simulink model "gpc_simulink"  (R2022a)
settings: Solver=VariableStepAuto  StartTime=0.0  StopTime=20  RelTol=1e-3
values from neighbouring files (symbols this model uses):
  H = inv(G'*G+lambda*eye(3))    [gpc.m]
  K = inv(G'*G+lambda*eye(3))*G'    [gpc.m]
  th = 1    [gpc.m]
undefined symbols (not defined in the file or in its folder): DiscIntNeverNeededParam
libraries: ctrlSharedLib x5, eeAlternativeControllers x1, slident x1
settings Model: Creator=mjwhi  LastModifiedBy=mjwhi

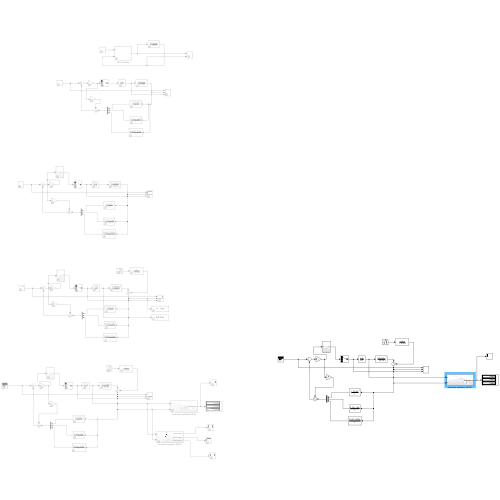
[thumbnail: Simulink's stored preview of the top-level diagram]
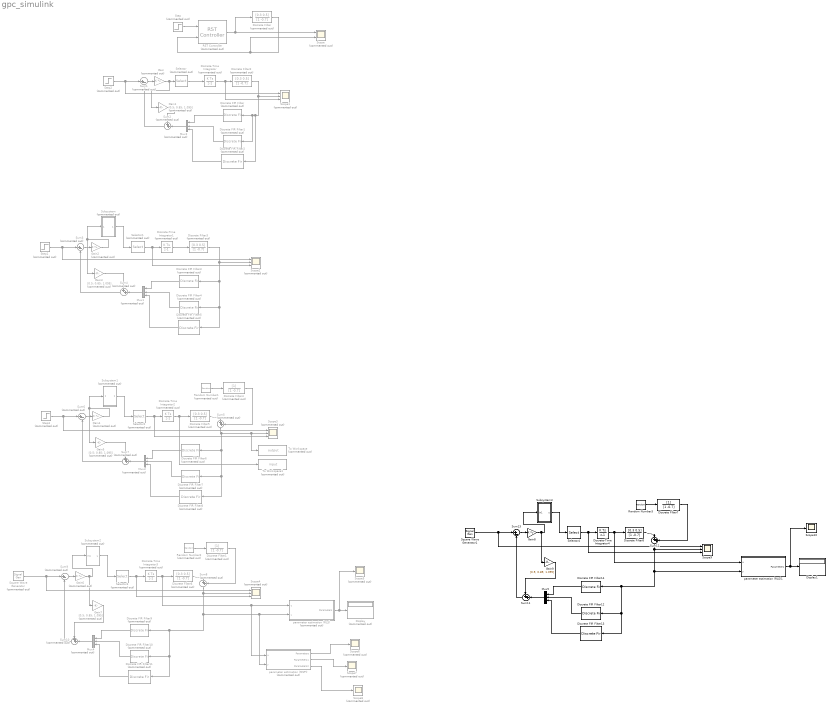
== system gpc_simulink ==
  Discrete FIR Filter{,3,6,9} (4 alike) : DiscreteFir  Commented=on  Coefficients=[1.7 -0.7]
  Discrete FIR Filter{1,4,7,10} (4 alike) : DiscreteFir  Commented=on  Coefficients=[2.19 -1.19]
  Discrete FIR Filter{2,5,8,11} (4 alike) : DiscreteFir  Commented=on  Coefficients=[2.533 -1.533]
  Discrete FIR Filter12 : DiscreteFir  Coefficients=[2.19 -1.19]
  Discrete FIR Filter13 : DiscreteFir  Coefficients=[2.533 -1.533]
  Discrete FIR Filter14 : DiscreteFir  Coefficients=[1.7 -0.7]
  Discrete Filter{,2..3,5} (4 alike) : DiscreteFilter  Commented=on  Numerator=[0.3 0.5]  Denominator=[1 -0.7]
  Discrete Filter1 : DiscreteFilter  Commented=on  Denominator=[1 -0.7]
  Discrete Filter4 : DiscreteFilter  Commented=on  Denominator=[1 -0.7]
  Discrete Filter6 : DiscreteFilter  Commented=on  Numerator=[0.3 0.5]  Denominator=[1 -0.7]  InitialStates=1
  Discrete Filter7 : DiscreteFilter  Denominator=[1 -0.7]
  Discrete Filter8 : DiscreteFilter  Numerator=[0.3 0.5]  Denominator=[1 -0.7]  InitialStates=1
  Discrete-Time Integrator{,1..3} (4 alike) : DiscreteIntegrator  Commented=on  SampleTime=-1  ICPrevOutput=DiscIntNeverNeededParam  ICPrevScaledInput=DiscIntNeverNeededParam
  Discrete-Time Integrator4 : DiscreteIntegrator  SampleTime=-1  ICPrevOutput=DiscIntNeverNeededParam  ICPrevScaledInput=DiscIntNeverNeededParam
  Display : Display  Commented=on
  Display1 : Display
  Gain{,2,4,6} (4 alike) : Gain  Commented=on  Gain=K  Multiplication=Matrix(K*u)
  Gain{1,3,5,7} (4 alike) : Gain  Commented=on  Gain=[0.5; 0.85; 1.095]
  Gain8 : Gain  Gain=K  Multiplication=Matrix(K*u)
  Gain9 : Gain  Gain=[0.5; 0.85; 1.095]
  Mux{1..4} (4 alike) : Mux  Commented=on  Inputs=3
  Mux5 : Mux  Inputs=3
  RST Controller : eeAlternativeControllers/RST Controller  Commented=on  CtrlParam=Generate polynomials  R=1  S=1  T=1  B=[0.3 0.5]  A=[1 -0.7]  N=3  lam=0.7  d=0  Ts=-1
      settings: SourceProductBaseCode=PS
  Random Number1 : RandomNumber  Commented=on  Variance=0.001  SampleTime=0.2
  Random Number2 : RandomNumber  Commented=on  Variance=0.001  SampleTime=0.2
  Random Number3 : RandomNumber  Variance=0.001  SampleTime=0.2
  Scope : Scope  Commented=on  NumInputPorts=2
  Scope{1..4} (4 alike) : Scope  Commented=on  NumInputPorts=3
  Scope10 : Scope
  Scope{5..8} (4 alike) : Scope  Commented=on
  Scope9 : Scope  NumInputPorts=3
  Selector{,1..3} (4 alike) : Selector  Commented=on  InputPortWidth=3  IndexOptions=Index vector (dialog)  Indices=[1]  OutputSizes=1
  Selector4 : Selector  InputPortWidth=3  IndexOptions=Index vector (dialog)  Indices=[1]  OutputSizes=1
  Square Wave Generator : SignalGenerator  Commented=on  WaveForm=square  Units=rad/sec
  Square Wave Generator1 : SignalGenerator  WaveForm=square  Units=rad/sec
  Step{,1..3} (4 alike) : Step  Commented=on  Time=0  SampleTime=0.2
  Subsystem : Subsystem  Commented=on
  Subsystem1 : Subsystem  Commented=on
  Subsystem2 : Subsystem  Commented=on
  Subsystem3 : Subsystem
  Sum{1,3,6,9} (4 alike) : Sum  Commented=on  Inputs=|+-
  Sum{2,4,7,10} (4 alike) : Sum  Commented=on  Inputs=++|
  Sum11 : Sum  Inputs=++|
  Sum12 : Sum  Inputs=|++
  Sum13 : Sum  Inputs=|+-
  Sum5 : Sum  Commented=on  Inputs=|++
  Sum8 : Sum  Commented=on  Inputs=|++
  To Workspace : ToWorkspace  Commented=on  VariableName=output  SaveFormat=Timeseries  SampleTime=-1
  To Workspace1 : ToWorkspace  Commented=on  VariableName=input  SaveFormat=Timeseries  SampleTime=-1
  parameter estimation (MSPI) : Subsystem  Commented=on
  parameter estimation (RLS) : Subsystem  Commented=on
  parameter estimation (RLS)1 : Subsystem
  wires:
  RST Controller/1 -> Discrete Filter/1, Scope/1
  Step/1 -> RST Controller/1
  Discrete Filter/1 -> Scope/2, RST Controller/2
  Sum1/1 -> Gain/1
  Sum2/1 -> Sum1/2
  Step2/1 -> Scope1/1, Sum1/1
  Gain/1 -> Gain1/1, Selector/1
  Gain1/1 -> Sum2/1
  Discrete Filter2/1 -> Discrete FIR Filter2/1, Discrete FIR Filter1/1, Discrete FIR Filter/1, Scope1/2
  Discrete FIR Filter/1 -> Mux2/1
  Discrete FIR Filter1/1 -> Mux2/2
  Discrete FIR Filter2/1 -> Mux2/3
  Mux2/1 -> Sum2/2
  Selector/1 -> Discrete-Time Integrator/1
  Discrete-Time Integrator/1 -> Scope1/3, Discrete Filter2/1
  Selector1/1 -> Scope2/3, Discrete-Time Integrator1/1
  Discrete-Time Integrator1/1 -> Discrete Filter3/1
  Mux1/1 -> Sum4/2
  Discrete FIR Filter5/1 -> Mux1/3
  Step1/1 -> Scope2/1, Sum3/1
  Gain3/1 -> Sum4/1
  Discrete FIR Filter3/1 -> Mux1/1
  Discrete FIR Filter4/1 -> Mux1/2
  Sum3/1 -> Gain2/1
  Gain2/1 -> Gain3/1, Subsystem/1(In1)
  Sum4/1 -> Sum3/2
  Subsystem/1(Out1) -> Selector1/1
  Discrete Filter3/1 -> Discrete FIR Filter4/1, Discrete FIR Filter5/1, Discrete FIR Filter3/1, Scope2/2
  Sum6/1 -> Gain4/1
  Discrete FIR Filter7/1 -> Mux3/2
  Discrete FIR Filter6/1 -> Mux3/1
  Discrete FIR Filter8/1 -> Mux3/3
  Gain5/1 -> Sum7/1
  Mux3/1 -> Sum7/2
  Step3/1 -> Scope3/1, Sum6/1
  Discrete-Time Integrator2/1 -> To Workspace1/1, Discrete Filter5/1
  Discrete Filter5/1 -> Sum5/1
  Sum7/1 -> Sum6/2
  Discrete Filter4/1 -> Sum5/2
  Sum5/1 -> Discrete FIR Filter7/1, Discrete FIR Filter8/1, Discrete FIR Filter6/1, Scope3/2, To Workspace/1
  Selector2/1 -> Scope3/3, Discrete-Time Integrator2/1
  Subsystem1/1(Out1) -> Selector2/1
  Random Number1/1 -> Discrete Filter4/1
  Gain4/1 -> Gain5/1, Subsystem1/1(In1)
  Subsystem2/1(u) -> Selector3/1
  Selector3/1 -> Scope4/3, Discrete-Time Integrator3/1
  Square Wave Generator/1 -> Scope4/1, Sum9/1
  Random Number2/1 -> Discrete Filter1/1
  Discrete-Time Integrator3/1 -> parameter estimation (RLS)/1(u), parameter estimation (MSPI)/1(u), Discrete Filter6/1
  Gain6/1 -> Gain7/1, Subsystem2/1(In1)
  Discrete Filter6/1 -> Sum8/1
  Sum9/1 -> Gain6/1
  Discrete Filter1/1 -> Sum8/2
  parameter estimation (RLS)/1(Parameters) -> Scope5/1, Display/1
  Sum8/1 -> Scope4/2, Discrete FIR Filter10/1, Discrete FIR Filter11/1, Discrete FIR Filter9/1, parameter estimation (RLS)/2(y), parameter estimation (MSPI)/2(y)
  Mux4/1 -> Sum10/2
  Sum10/1 -> Sum9/2
  Discrete FIR Filter11/1 -> Mux4/3
  Gain7/1 -> Sum10/1
  Discrete FIR Filter9/1 -> Mux4/1
  Discrete FIR Filter10/1 -> Mux4/2
  parameter estimation (MSPI)/1(Parameters) -> Scope6/1
  parameter estimation (MSPI)/2(Parameters1) -> Scope7/1
  parameter estimation (MSPI)/3(Parameters2) -> Scope8/1
  Sum11/1 -> Sum13/2
  Discrete FIR Filter14/1 -> Mux5/1
  Discrete FIR Filter12/1 -> Mux5/2
  Mux5/1 -> Sum11/2
  parameter estimation (RLS)1/1(Parameters) -> Scope10/1, Display1/1
  Gain9/1 -> Sum11/1
  Sum12/1 -> Scope9/2, Discrete FIR Filter12/1, Discrete FIR Filter13/1, Discrete FIR Filter14/1, parameter estimation (RLS)1/2(y)
  Discrete Filter7/1 -> Sum12/2
  Gain8/1 -> Gain9/1, Subsystem3/1(In1)
  Discrete-Time Integrator4/1 -> parameter estimation (RLS)1/1(u), Discrete Filter8/1
  Discrete FIR Filter13/1 -> Mux5/3
  Random Number3/1 -> Discrete Filter7/1
  Sum13/1 -> Gain8/1
  Discrete Filter8/1 -> Sum12/1
  Square Wave Generator1/1 -> Scope9/1, Sum13/1
  Subsystem3/1(u) -> Selector4/1
  Selector4/1 -> Scope9/3, Discrete-Time Integrator4/1

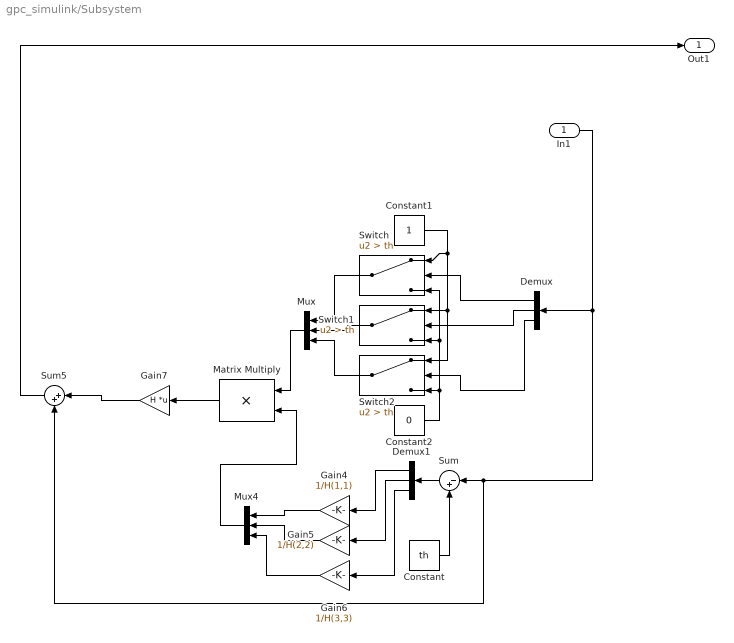
== system gpc_simulink/Subsystem ==
  In1 : Inport
  Constant : Constant  Value=th
  Constant1 : Constant
  Constant2 : Constant  Value=0
  Demux : Demux  Outputs=3
  Demux1 : Demux  Outputs=3
  Gain4 : Gain  Gain=1/H(1,1)
  Gain5 : Gain  Gain=1/H(2,2)
  Gain6 : Gain  Gain=1/H(3,3)
  Gain7 : Gain  Gain=H  Multiplication=Matrix(K*u)
  Matrix Multiply : Product
  Mux : Mux  Inputs=3
  Mux4 : Mux  Inputs=3
  Sum : Sum  Inputs=|-+
  Sum5 : Sum  Inputs=|++
  Switch : Switch  Criteria=u2 > Threshold  Threshold=th  SaturateOnIntegerOverflow=off  InputSameDT=off
  Switch1 : Switch  Criteria=u2 > Threshold  Threshold=th  SaturateOnIntegerOverflow=off  InputSameDT=off
  Switch2 : Switch  Criteria=u2 > Threshold  Threshold=th  SaturateOnIntegerOverflow=off  InputSameDT=off
  Out1 : Outport
  wires:
  Mux4/1 -> Matrix Multiply/2
  Demux/3 -> Switch2/2
  Constant2/1 -> Switch/3, Switch1/3, Switch2/3
  In1/1 -> Sum5/2, Sum/1, Demux/1
  Mux/1 -> Matrix Multiply/1
  Constant1/1 -> Switch/1, Switch2/1, Switch1/1
  Sum/1 -> Demux1/1
  Gain4/1 -> Mux4/1
  Demux1/3 -> Gain6/1
  Constant/1 -> Sum/2
  Gain7/1 -> Sum5/1
  Demux/1 -> Switch/2
  Gain5/1 -> Mux4/2
  Demux/2 -> Switch1/2
  Matrix Multiply/1 -> Gain7/1
  Switch/1 -> Mux/1
  Switch1/1 -> Mux/2
  Demux1/2 -> Gain5/1
  Switch2/1 -> Mux/3
  Demux1/1 -> Gain4/1
  Gain6/1 -> Mux4/3
  Sum5/1 -> Out1/1

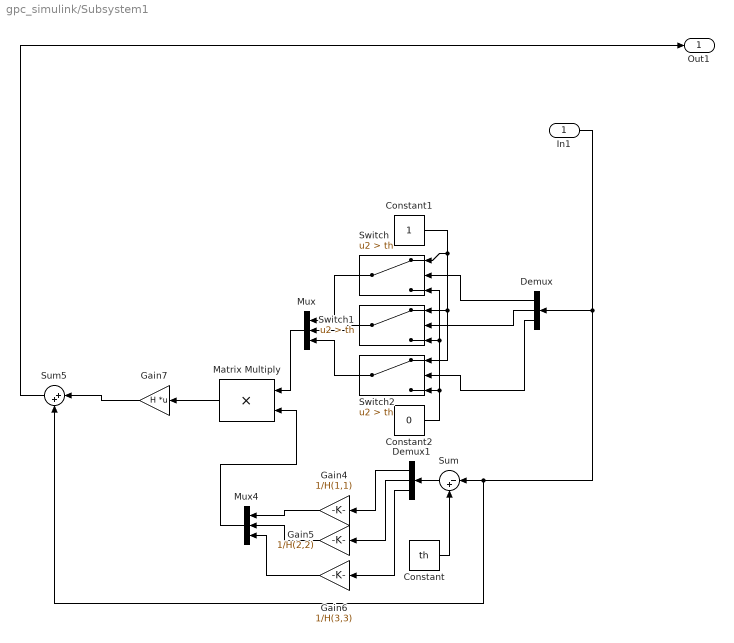
== system gpc_simulink/Subsystem1 ==
  In1 : Inport
  Constant : Constant  Value=th
  Constant1 : Constant
  Constant2 : Constant  Value=0
  Demux : Demux  Outputs=3
  Demux1 : Demux  Outputs=3
  Gain4 : Gain  Gain=1/H(1,1)
  Gain5 : Gain  Gain=1/H(2,2)
  Gain6 : Gain  Gain=1/H(3,3)
  Gain7 : Gain  Gain=H  Multiplication=Matrix(K*u)
  Matrix Multiply : Product
  Mux : Mux  Inputs=3
  Mux4 : Mux  Inputs=3
  Sum : Sum  Inputs=|-+
  Sum5 : Sum  Inputs=|++
  Switch : Switch  Criteria=u2 > Threshold  Threshold=th  SaturateOnIntegerOverflow=off  InputSameDT=off
  Switch1 : Switch  Criteria=u2 > Threshold  Threshold=th  SaturateOnIntegerOverflow=off  InputSameDT=off
  Switch2 : Switch  Criteria=u2 > Threshold  Threshold=th  SaturateOnIntegerOverflow=off  InputSameDT=off
  Out1 : Outport
  wires:
  Mux4/1 -> Matrix Multiply/2
  Demux/3 -> Switch2/2
  Constant2/1 -> Switch/3, Switch1/3, Switch2/3
  In1/1 -> Sum5/2, Sum/1, Demux/1
  Mux/1 -> Matrix Multiply/1
  Constant1/1 -> Switch/1, Switch2/1, Switch1/1
  Sum/1 -> Demux1/1
  Gain4/1 -> Mux4/1
  Demux1/3 -> Gain6/1
  Constant/1 -> Sum/2
  Gain7/1 -> Sum5/1
  Demux/1 -> Switch/2
  Gain5/1 -> Mux4/2
  Demux/2 -> Switch1/2
  Matrix Multiply/1 -> Gain7/1
  Switch/1 -> Mux/1
  Switch1/1 -> Mux/2
  Demux1/2 -> Gain5/1
  Switch2/1 -> Mux/3
  Demux1/1 -> Gain4/1
  Gain6/1 -> Mux4/3
  Sum5/1 -> Out1/1

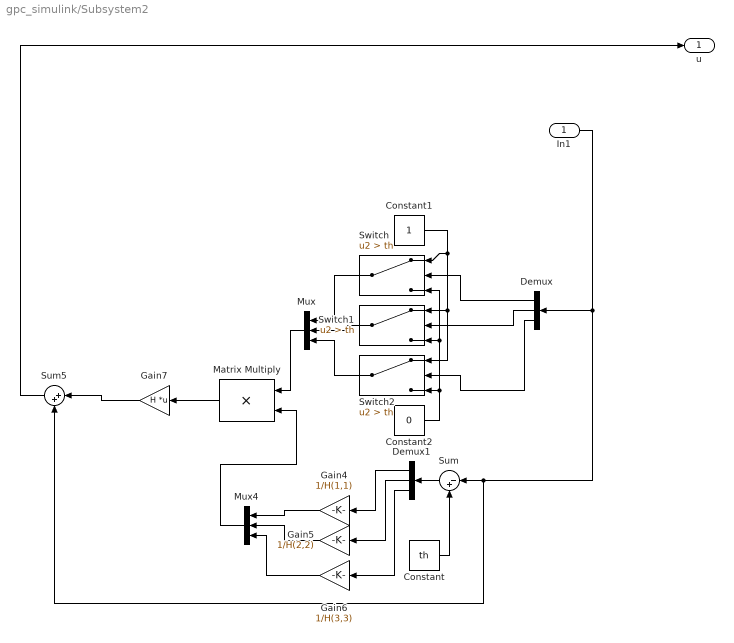
== system gpc_simulink/Subsystem2 ==
  In1 : Inport
  Constant : Constant  Value=th
  Constant1 : Constant
  Constant2 : Constant  Value=0
  Demux : Demux  Outputs=3
  Demux1 : Demux  Outputs=3
  Gain4 : Gain  Gain=1/H(1,1)
  Gain5 : Gain  Gain=1/H(2,2)
  Gain6 : Gain  Gain=1/H(3,3)
  Gain7 : Gain  Gain=H  Multiplication=Matrix(K*u)
  Matrix Multiply : Product
  Mux : Mux  Inputs=3
  Mux4 : Mux  Inputs=3
  Sum : Sum  Inputs=|-+
  Sum5 : Sum  Inputs=|++
  Switch : Switch  Criteria=u2 > Threshold  Threshold=th  SaturateOnIntegerOverflow=off  InputSameDT=off
  Switch1 : Switch  Criteria=u2 > Threshold  Threshold=th  SaturateOnIntegerOverflow=off  InputSameDT=off
  Switch2 : Switch  Criteria=u2 > Threshold  Threshold=th  SaturateOnIntegerOverflow=off  InputSameDT=off
  u : Outport
  wires:
  Mux4/1 -> Matrix Multiply/2
  Demux/3 -> Switch2/2
  Constant2/1 -> Switch/3, Switch1/3, Switch2/3
  In1/1 -> Sum5/2, Sum/1, Demux/1
  Mux/1 -> Matrix Multiply/1
  Constant1/1 -> Switch/1, Switch2/1, Switch1/1
  Sum/1 -> Demux1/1
  Gain4/1 -> Mux4/1
  Demux1/3 -> Gain6/1
  Constant/1 -> Sum/2
  Gain7/1 -> Sum5/1
  Demux/1 -> Switch/2
  Gain5/1 -> Mux4/2
  Demux/2 -> Switch1/2
  Matrix Multiply/1 -> Gain7/1
  Switch/1 -> Mux/1
  Switch1/1 -> Mux/2
  Demux1/2 -> Gain5/1
  Switch2/1 -> Mux/3
  Demux1/1 -> Gain4/1
  Gain6/1 -> Mux4/3
  Sum5/1 -> u/1

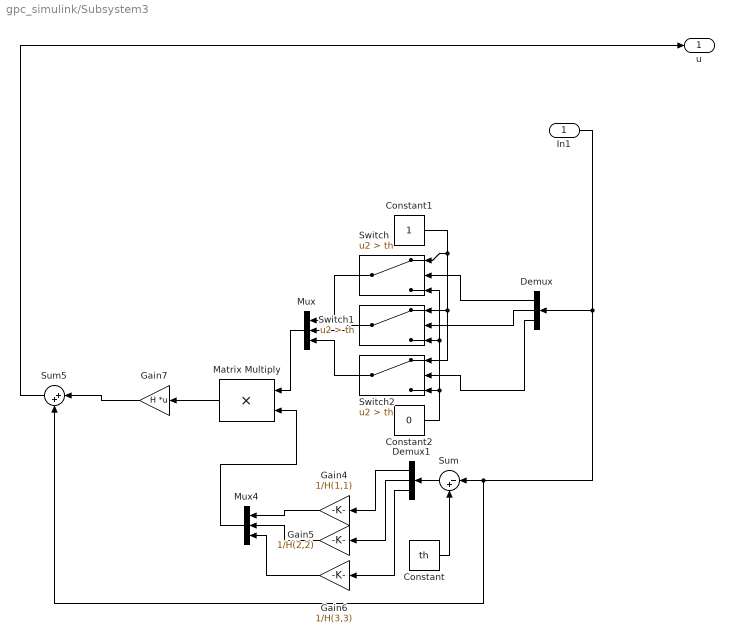
== system gpc_simulink/Subsystem3 ==
  In1 : Inport
  Constant : Constant  Value=th
  Constant1 : Constant
  Constant2 : Constant  Value=0
  Demux : Demux  Outputs=3
  Demux1 : Demux  Outputs=3
  Gain4 : Gain  Gain=1/H(1,1)
  Gain5 : Gain  Gain=1/H(2,2)
  Gain6 : Gain  Gain=1/H(3,3)
  Gain7 : Gain  Gain=H  Multiplication=Matrix(K*u)
  Matrix Multiply : Product
  Mux : Mux  Inputs=3
  Mux4 : Mux  Inputs=3
  Sum : Sum  Inputs=|-+
  Sum5 : Sum  Inputs=|++
  Switch : Switch  Criteria=u2 > Threshold  Threshold=th  SaturateOnIntegerOverflow=off  InputSameDT=off
  Switch1 : Switch  Criteria=u2 > Threshold  Threshold=th  SaturateOnIntegerOverflow=off  InputSameDT=off
  Switch2 : Switch  Criteria=u2 > Threshold  Threshold=th  SaturateOnIntegerOverflow=off  InputSameDT=off
  u : Outport
  wires:
  Mux4/1 -> Matrix Multiply/2
  Demux/3 -> Switch2/2
  Constant2/1 -> Switch/3, Switch1/3, Switch2/3
  In1/1 -> Sum5/2, Sum/1, Demux/1
  Mux/1 -> Matrix Multiply/1
  Constant1/1 -> Switch/1, Switch2/1, Switch1/1
  Sum/1 -> Demux1/1
  Gain4/1 -> Mux4/1
  Demux1/3 -> Gain6/1
  Constant/1 -> Sum/2
  Gain7/1 -> Sum5/1
  Demux/1 -> Switch/2
  Gain5/1 -> Mux4/2
  Demux/2 -> Switch1/2
  Matrix Multiply/1 -> Gain7/1
  Switch/1 -> Mux/1
  Switch1/1 -> Mux/2
  Demux1/2 -> Gain5/1
  Switch2/1 -> Mux/3
  Demux1/1 -> Gain4/1
  Gain6/1 -> Mux4/3
  Sum5/1 -> u/1

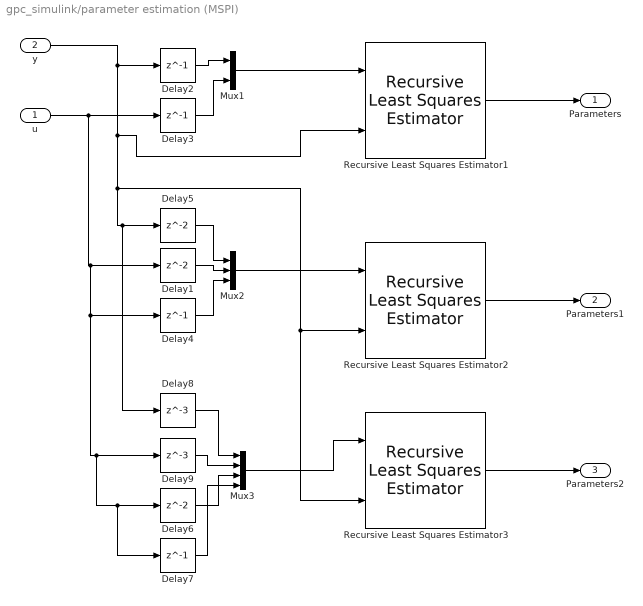
== system gpc_simulink/parameter estimation (MSPI) ==
  u : Inport
  y : Inport  Port=2
  Delay1 : Delay
  Delay{2..4,7} (4 alike) : Delay  DelayLength=1
  Delay5 : Delay
  Delay6 : Delay
  Delay8 : Delay  DelayLength=3
  Delay9 : Delay  DelayLength=3
  Mux1 : Mux  Inputs=2
  Mux2 : Mux  Inputs=3
  Mux3 : Mux
  Recursive Least Squares Estimator1 : ctrlSharedLib/Recursive Least Squares Estimator  InitialEstimateSource=Internal  InitialParameterData=[0 0]  P0=1e4  InitialRegressors=0  InitialOutputs=0  History=Infinite  WindowLength=200  EstimationMethod=Kalman Filter  AdaptationParameter=0  HasTimeVaryingAdaptationParameter=off  NormalizationBias=eps  OutputError=off  OutputP=off  AddEnablePort=off  InputProcessing=Sample-based  Ts=-1
      settings: SourceProductBaseCode=CT,ID
  Recursive Least Squares Estimator2 : ctrlSharedLib/Recursive Least Squares Estimator  InitialEstimateSource=Internal  InitialParameterData=[0 0 0]  P0=1e4  InitialRegressors=0  InitialOutputs=0  History=Infinite  WindowLength=200  EstimationMethod=Kalman Filter  AdaptationParameter=0  HasTimeVaryingAdaptationParameter=off  NormalizationBias=eps  OutputError=off  OutputP=off  AddEnablePort=off  InputProcessing=Sample-based  Ts=-1
      settings: SourceProductBaseCode=CT,ID
  Recursive Least Squares Estimator3 : ctrlSharedLib/Recursive Least Squares Estimator  InitialEstimateSource=Internal  InitialParameterData=[0 0 0 0]  P0=1e4  InitialRegressors=0  InitialOutputs=0  History=Infinite  WindowLength=200  EstimationMethod=Kalman Filter  AdaptationParameter=0  HasTimeVaryingAdaptationParameter=off  NormalizationBias=eps  OutputError=off  OutputP=off  AddEnablePort=off  InputProcessing=Sample-based  Ts=-1
      settings: SourceProductBaseCode=CT,ID
  Parameters : Outport
  Parameters1 : Outport  Port=2
  Parameters2 : Outport  Port=3
  wires:
  y/1 -> Delay2/1, Recursive Least Squares Estimator3/2, Recursive Least Squares Estimator2/2, Delay8/1, Delay5/1, Recursive Least Squares Estimator1/2
  Delay2/1 -> Mux1/1
  Delay3/1 -> Mux1/2
  Mux1/1 -> Recursive Least Squares Estimator1/1
  Recursive Least Squares Estimator1/1 -> Parameters/1
  Delay4/1 -> Mux2/3
  Delay1/1 -> Mux2/2
  Mux2/1 -> Recursive Least Squares Estimator2/1
  Recursive Least Squares Estimator2/1 -> Parameters1/1
  u/1 -> Delay7/1, Delay6/1, Delay9/1, Delay4/1, Delay1/1, Delay3/1
  Delay5/1 -> Mux2/1
  Recursive Least Squares Estimator3/1 -> Parameters2/1
  Delay8/1 -> Mux3/1
  Delay9/1 -> Mux3/2
  Delay6/1 -> Mux3/3
  Delay7/1 -> Mux3/4
  Mux3/1 -> Recursive Least Squares Estimator3/1

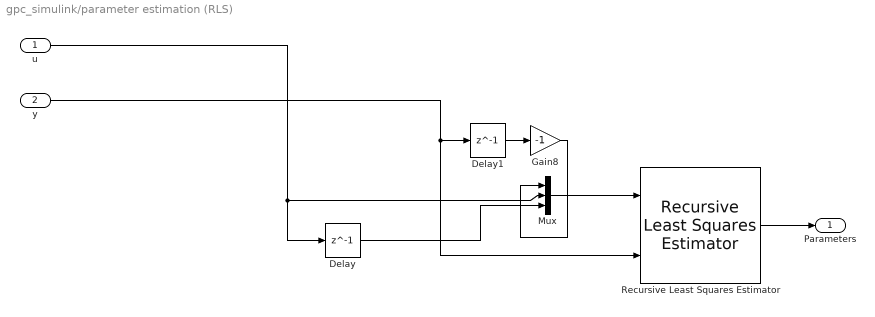
== system gpc_simulink/parameter estimation (RLS) ==
  u : Inport
  y : Inport  Port=2
  Delay : Delay  DelayLength=1
  Delay1 : Delay  DelayLength=1
  Gain8 : Gain  Gain=-1
  Mux : Mux  Inputs=3
  Recursive Least Squares Estimator : ctrlSharedLib/Recursive Least Squares Estimator  InitialEstimateSource=Internal  InitialParameterData=[-0.6 0.2 0.6]  P0=1e4  InitialRegressors=0  InitialOutputs=0  History=Infinite  WindowLength=200  EstimationMethod=Kalman Filter  AdaptationParameter=0  HasTimeVaryingAdaptationParameter=off  NormalizationBias=eps  OutputError=off  OutputP=off  AddEnablePort=off  InputProcessing=Sample-based  Ts=-1
      settings: SourceProductBaseCode=CT,ID
  Parameters : Outport
  wires:
  Delay/1 -> Mux/3
  u/1 -> Mux/2, Delay/1
  Delay1/1 -> Gain8/1
  Mux/1 -> Recursive Least Squares Estimator/1
  Gain8/1 -> Mux/1
  Recursive Least Squares Estimator/1 -> Parameters/1
  y/1 -> Recursive Least Squares Estimator/2, Delay1/1

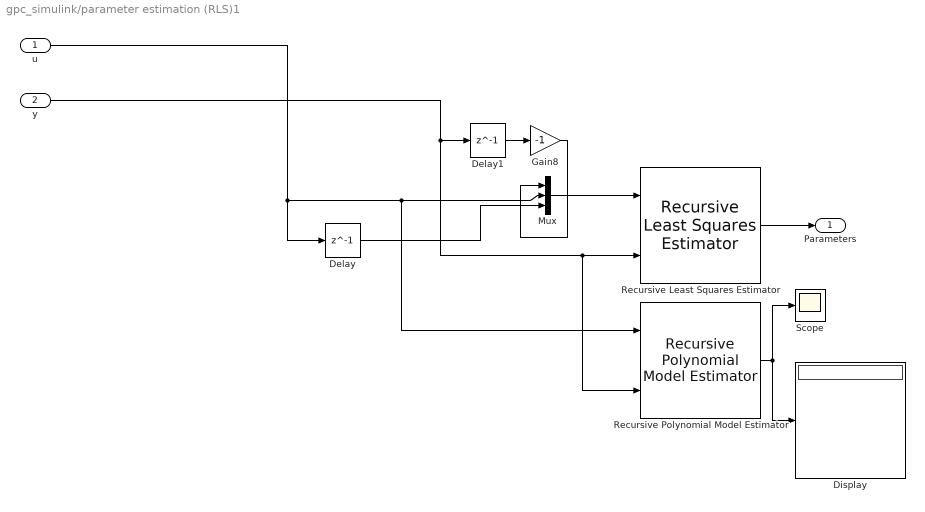
== system gpc_simulink/parameter estimation (RLS)1 ==
  u : Inport
  y : Inport  Port=2
  Delay : Delay  DelayLength=1
  Delay1 : Delay  DelayLength=1
  Display : Display
  Gain8 : Gain  Gain=-1
  Mux : Mux  Inputs=3
  Recursive Least Squares Estimator : ctrlSharedLib/Recursive Least Squares Estimator  InitialEstimateSource=Internal  InitialParameterData=[-0.6 0.2 0.6]  P0=1e4  InitialRegressors=0  InitialOutputs=0  History=Infinite  WindowLength=200  EstimationMethod=Kalman Filter  AdaptationParameter=0  HasTimeVaryingAdaptationParameter=off  NormalizationBias=eps  OutputError=off  OutputP=off  AddEnablePort=off  InputProcessing=Sample-based  Ts=-1
      settings: SourceProductBaseCode=CT,ID
  Recursive Polynomial Model Estimator : slident/Estimators/Recursive Polynomial Model Estimator  ModelStructure=ARX  InitialEstimateSource=Internal  A0=[1 -0.6]  B0=[0.2 0.6]  C0=1  D0=1  F0=1  nk=1  P0=1e4  InitialInputs=0  InitialOutputs=0  History=Infinite  WindowLength=200  EstimationMethod=Forgetting Factor  AdaptationParameter=1  HasTimeVaryingAdaptationParameter=off  NormalizationBias=eps  OutputError=off  OutputP=off  AddEnablePort=off  InputProcessing=Sample-based  Ts=-1
      settings: SourceProductBaseCode=ID
  Scope : Scope
  Parameters : Outport
  wires:
  Delay/1 -> Mux/3
  u/1 -> Recursive Polynomial Model Estimator/1, Mux/2, Delay/1
  Delay1/1 -> Gain8/1
  Mux/1 -> Recursive Least Squares Estimator/1
  Gain8/1 -> Mux/1
  Recursive Least Squares Estimator/1 -> Parameters/1
  y/1 -> Recursive Polynomial Model Estimator/2, Recursive Least Squares Estimator/2, Delay1/1
  Recursive Polynomial Model Estimator/1 -> Scope/1, Display/1
